simulink model "suspension"  (R2018a)
settings: Solver=VariableStepAuto  StartTime=0.0  StopTime=50  RelTol=1e-3
values from neighbouring files (symbols this model uses):
  b1 = 350    [start.m]
  b2 = 15020    [start.m]
  K1 = 80000    [start.m]
  K2 = 500000    [start.m]
  M1 = 2500    [start.m]
  M2 = 320    [start.m]
libraries: simulink x1
settings Model: Creator=maroufi  LastModifiedBy=maroufi

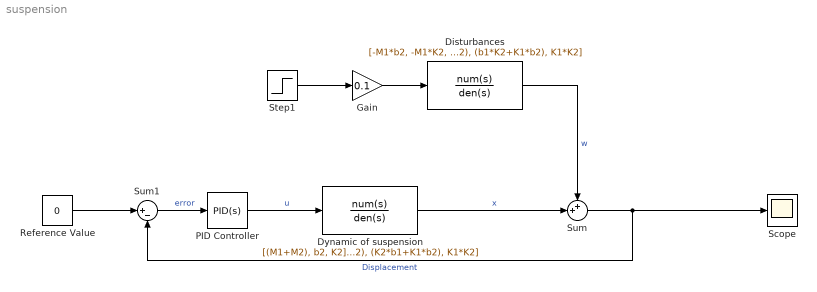
== system suspension ==
  Disturbances : TransferFcn  Numerator=[-M1*b2, -M1*K2, 0, 0]  Denominator=[M1*M2, (M1*b1+M1*b2+M2*b1), (M1*K1+M1*K2+b1*b2+K1*M2), (b1*K2+K1*b2), K1*K2]
  Dynamic of suspension : TransferFcn  Numerator=[(M1+M2), b2, K2]  Denominator=[M1*M2, (M1*b1+M1*b2+M2*b1), (M1*K1+M1*K2+b1*b2+K1*M2), (K2*b1+K1*b2), K1*K2]
  Gain : Gain  Gain=0.1
  PID Controller : simulink/Continuous/PID Controller  Controller=PID  TimeDomain=Continuous-time  SampleTime=-1  IntegratorMethod=Forward Euler  FilterMethod=Forward Euler  Form=Parallel  UseFilter=on  ControllerParametersSource=internal  P=90000  I=1  D=0  N=100  InitialConditionSource=internal  InitialConditionForIntegrator=0  InitialConditionForFilter=0  ExternalReset=none  LimitOutput=off  UpperSaturationLimit=inf  LowerSaturationLimit=-inf  LinearizeAsGain=on  AntiWindupMode=none  Kb=1  TrackingMode=off  Kt=1  PParamMin=[]  PParamMax=[]  IParamMin=[]  IParamMax=[]  DParamMin=[]  DParamMax=[]  NParamMin=[]  NParamMax=[]  KbParamMin=[]  KbParamMax=[]  KtParamMin=[]  KtParamMax=[]  POutMin=[]  POutMax=[]  IOutMin=[]  IOutMax=[]  DOutMin=[]  DOutMax=[]  NOutMin=[]  NOutMax=[]  KbOutMin=[]  KbOutMax=[]  KtOutMin=[]  KtOutMax=[]  IntegratorOutMin=[]  IntegratorOutMax=[]  FilterOutMin=[]  FilterOutMax=[]  SumOutMin=[]  SumOutMax=[]  SumI1OutMin=[]  SumI1OutMax=[]  SumI2OutMin=[]  SumI2OutMax=[]  SumI3OutMin=[]  SumI3OutMax=[]  SumDOutMin=[]  SumDOutMax=[]  SaturationOutMin=[]  SaturationOutMax=[]  IntegratorContinuousStateAttributes=''  IntegratorStateMustResolveToSignalObject=off  IntegratorRTWStateStorageClass=Auto  FilterContinuousStateAttributes=''  FilterStateMustResolveToSignalObject=off  FilterRTWStateStorageClass=Auto  DifferentiatorICPrevScaledInput=0  DifferentiatorOutMin=[]  DifferentiatorOutMax=[]  FilterDiffOutCoefMin=[]  FilterDiffOutCoefMax=[]  SumDenOutMin=[]  SumDenOutMax=[]  SumNumOutMin=[]  SumNumOutMax=[]  ReciprocalOutMin=[]  ReciprocalOutMax=[]  DivideOutMin=[]  DivideOutMax=[]  TunerSelectOption=Transfer Function Based (PID Tuner App)
  Reference Value : Constant  Value=0
  Scope : Scope
  Step1 : Step  SampleTime=0
  Sum : Sum  Inputs=++|
  Sum1 : Sum  Inputs=|+-
  wires:
  PID Controller/1 -> Dynamic of suspension/1  "u"
  Dynamic of suspension/1 -> Sum/2  "x"
  Step1/1 -> Gain/1
  Gain/1 -> Disturbances/1
  Disturbances/1 -> Sum/1  "w"
  Sum/1 -> Sum1/2, Scope/1  "Displacement"
  Sum1/1 -> PID Controller/1  "error"
  Reference Value/1 -> Sum1/1
